simulink model "modulation_cosim"  (Simulink 7.0)
settings: Solver=FixedStepDiscrete  StartTime=0.0  StopTime=10.0  RelTol=1e-3
undefined symbols (not defined in the file): image, port_label
libraries: aldec_ahdl x5
settings Model: Creator=arekg  LastModifiedBy=arekg
settings DataIOCC: SignalLoggingName=sigsOut
settings OptimizationCC: InlineInvariantSignals=on
settings DebuggingCC: SaveWithParameterizedLinksMsg=none  SignalResolutionControl=TryResolveAllWithWarning  SolverPrmCheckMsg=none  MultiTaskDSMMsg=warning  MultiTaskCondExecSysMsg=none
settings HardwareCC: TargetUnknown=on
settings RTWCC: IncludeERTFirstTime=on
settings GRTTargetCC: TargetFcnLib=ansi_tfl_tmw.mat  ModelReferenceCompliant=off  MatFileLogging=off

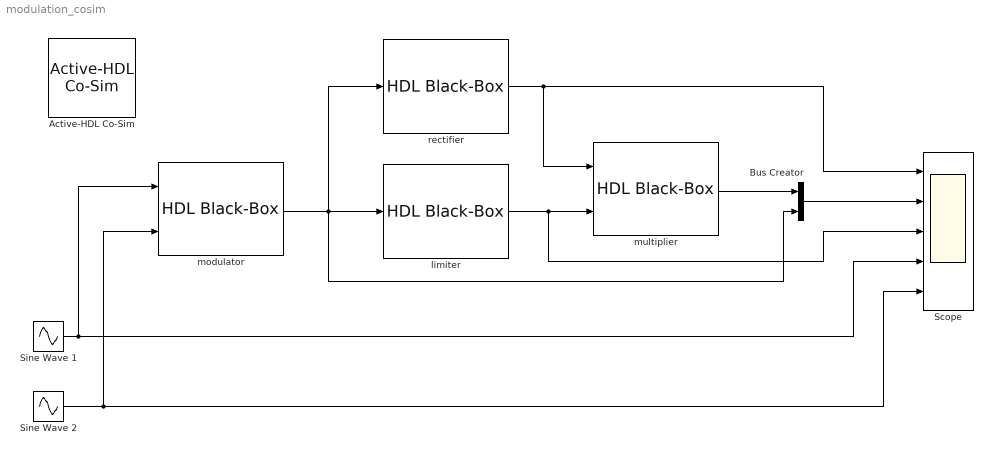
== system modulation_cosim ==
  Active-HDL Co-Sim : aldec_ahdl/Active-HDL Co-Sim  Tag=Active-HDL_Co-Sim_close  hdl_period=1/20  hdl_tscale=sec  sys_period=[1/20, 0]  sys_tscale=As In Simulator  wav_fn=mlab_cosim  wav_settings=[0,0,0,0,0,0,0,0]  dbg=off  auto_start=off  gen_tb=[0,0]  batch_sim=off  tb_fn=mlab_post_tb.log  metavalue_map=[0,0]  sim_resolution=[1,0,0]  active_page=0  aws_en=off  ahdl_en=off  blk_ver=9.1.RTM  macro_en=[1,0,1]  macro_path=prepare_project.do  mfun_text=check_mfiles
  Bus Creator : BusCreator  Inputs=2
  Scope : Scope  NumInputPorts=5
      settings: YMin=-1~-40~-2~-1~-1.5  YMax=40~40~2~40~1.5
  Sine Wave 1 : Sin  Amplitude=18  Bias=20  Frequency=0.5*pi  Phase=pi/1.3  SampleTime=1/20
  Sine Wave 2 : Sin  Amplitude=0.9  Frequency=pi/0.4  Phase=pi  SampleTime=1/20
  limiter : aldec_ahdl/HDL Black-Box  module_m=signum  ports_cfg={In1,0,31,0,24,1,0,0,0,0,0,0}{Out1,1,2,0,0,1,0,0,0,0,0,0}  hdl_src=c:\My_Designs\Samples_73\simulink_example\Modulation\src\sign.vhd  block_mask=image(imread('HDLBlackBox.jpg'),'center'); disp('signum');port_label('input', 1, 'In1');port_label('output', 1, 'Out1');  config=[1,1]  inp=[1, 0, 31, 24, 0, 0, 0]  out=[1, 0, 2, 0, 0, 0, 0]  sampling=[0,1,1]  active_page={0}{80,0,35,1,65,2,70,3,70,4,60,5,60,6,50,7,35,8,35,9,119,10}{103,0,55,1,70,2,75,3,75,4,45,5,45,6,45,7,165,8,0,0,0,0}{165,0,130,1,190,2,190,3,0,0,0,0,0,0,0,0,0,0,0,0,0,0}{81,0,60,1,60,2,70,3,60,4,0,0,0,0,0,0,0,0,0,0,0,0}{83,0,70,1,80,2,50,3,50,4,0,0,0,0,0,0,0,0,0,0,0,0}{125,0,330,1,220,2,0,0,0,0,0,0,0,0,0,0,0,0,0,0,0,0}{95,0,95,1,70,2,50,3,80,4,35,5,35,6,65,7,150,8,0,0,0,0}{735,436}  param_val=0  clk_val=[0]  ce_val=[0]  blk_ver=9.1.RTM  blk_conf=0  user_conv=0
  modulator : aldec_ahdl/HDL Black-Box  module_m=mult  ports_cfg={Sin_wav1,0,16,0,9,1,0,0,0,0,0,0}{Sin_wav2,0,16,0,15,1,0,0,0,0,0,0}{Out1,1,31,0,24,1,0,0,0,0,0,0}  hdl_src=c:\My_Designs\Samples_73\simulink_example\Modulation\src\mult.vhd  block_mask=image(imread('HDLBlackBox.jpg'),'center'); disp('mult');port_label('input', 1, 'Sin_wav1');port_label('input', 2, 'Sin_wav2');port_label('output', 1, 'Out1');  config=[2,1]  inp=[2, 0, 16, 9, 0, 0, 0, 0, 16, 15, 0, 0, 0]  out=[1, 0, 31, 24, 0, 0, 0]  sampling=[0,1,1,1]  active_page={0}{80,0,35,1,65,2,70,3,70,4,60,5,60,6,50,7,35,8,35,9,119,10}{103,0,55,1,70,2,75,3,75,4,45,5,45,6,45,7,165,8,0,0,0,0}{165,0,130,1,190,2,190,3,0,0,0,0,0,0,0,0,0,0,0,0,0,0}{81,0,60,1,60,2,70,3,60,4,0,0,0,0,0,0,0,0,0,0,0,0}{83,0,70,1,80,2,50,3,50,4,0,0,0,0,0,0,0,0,0,0,0,0}{125,0,330,1,220,2,0,0,0,0,0,0,0,0,0,0,0,0,0,0,0,0}{95,0,95,1,70,2,50,3,80,4,35,5,35,6,65,7,150,8,0,0,0,0}{735,436}  param_val=0  clk_val=[0]  ce_val=[0]  blk_ver=9.1.RTM  blk_conf=0  user_conv=0
  multiplier : aldec_ahdl/HDL Black-Box  module_m=mult1  ports_cfg={I_abs,0,31,0,24,1,0,0,0,0,0,0}{I_sig,0,2,0,0,1,0,0,0,0,0,0}{Out1,1,31,0,24,1,0,0,0,0,0,0}  hdl_src=c:\My_Designs\Samples_73\simulink_example\Modulation\src\mult1.vhd  block_mask=image(imread('HDLBlackBox.jpg'),'center'); disp('mult1');port_label('input', 1, 'I_abs');port_label('input', 2, 'I_sig');port_label('output', 1, 'Out1');  config=[2,1]  inp=[2, 0, 31, 24, 0, 0, 0, 0, 2, 0, 0, 0, 0]  out=[1, 0, 31, 24, 0, 0, 0]  sampling=[0,1,1,1]  active_page={0}{80,0,35,1,65,2,70,3,70,4,60,5,60,6,50,7,35,8,35,9,119,10}{103,0,55,1,70,2,75,3,75,4,45,5,45,6,45,7,165,8,0,0,0,0}{165,0,130,1,190,2,190,3,0,0,0,0,0,0,0,0,0,0,0,0,0,0}{81,0,60,1,60,2,70,3,60,4,0,0,0,0,0,0,0,0,0,0,0,0}{83,0,70,1,80,2,50,3,50,4,0,0,0,0,0,0,0,0,0,0,0,0}{125,0,330,1,220,2,0,0,0,0,0,0,0,0,0,0,0,0,0,0,0,0}{95,0,95,1,70,2,50,3,80,4,35,5,35,6,65,7,150,8,0,0,0,0}{735,436}  param_val=0  clk_val=[0]  ce_val=[0]  blk_ver=9.1.RTM  blk_conf=0  user_conv=0
  rectifier : aldec_ahdl/HDL Black-Box  module_m=m_abs  ports_cfg={In1,0,31,0,24,1,0,0,0,0,0,0}{Out1,1,31,0,24,1,0,0,0,0,0,0}  hdl_src=c:\My_Designs\Samples_73\simulink_example\Modulation\src\abs.vhd  block_mask=image(imread('HDLBlackBox.jpg'),'center'); disp('m_abs');port_label('input', 1, 'In1');port_label('output', 1, 'Out1');  config=[1,1]  inp=[1, 0, 31, 24, 0, 0, 0]  out=[1, 0, 31, 24, 0, 0, 0]  sampling=[0,1,1]  active_page={0}{80,0,35,1,65,2,70,3,70,4,60,5,60,6,50,7,35,8,35,9,119,10}{103,0,55,1,70,2,75,3,75,4,45,5,45,6,45,7,165,8,0,0,0,0}{165,0,130,1,190,2,190,3,0,0,0,0,0,0,0,0,0,0,0,0,0,0}{81,0,60,1,60,2,70,3,60,4,0,0,0,0,0,0,0,0,0,0,0,0}{83,0,70,1,80,2,50,3,50,4,0,0,0,0,0,0,0,0,0,0,0,0}{125,0,330,1,220,2,0,0,0,0,0,0,0,0,0,0,0,0,0,0,0,0}{95,0,95,1,70,2,50,3,80,4,35,5,35,6,65,7,150,8,0,0,0,0}{735,436}  param_val=0  clk_val=[0]  ce_val=[0]  blk_ver=9.1.RTM  blk_conf=0  user_conv=0
  wires:
  rectifier/1 -> Scope/1, multiplier/1
  Sine Wave 1/1 -> Scope/4, modulator/1
  Sine Wave 2/1 -> Scope/5, modulator/2
  modulator/1 -> Bus Creator/2, limiter/1, rectifier/1
  limiter/1 -> Scope/3, multiplier/2
  multiplier/1 -> Bus Creator/1
  Bus Creator/1 -> Scope/2
